simulink model "VCU10"  (R2021b)
settings: Solver=FixedStepDiscrete  StartTime=0.0  StopTime=10.0  FixedStep=0.01  RelTol=1e-3
undefined symbols (not defined in the file): F, T
libraries: simulink x149, hdlsllib x90, spsEdgeDetectorLib x2
(part 1 of 3)
settings Model: DataDictionary=VCU10DB.sldd  Creator=icemi  LastModifiedBy=icemi
settings OptimizationCC: DefaultParameterBehavior=Inlined  EnhancedBackFolding=on  PassReuseOutputArgsAs=Individual arguments  ZeroExternalMemoryAtStartup=off  ZeroInternalMemoryAtStartup=off  OptimizeBlockOrder=speed  DifferentSizesBufferReuse=on  OptimizationCustomize=off  EfficientTunableParamExpr=on
settings DebuggingCC: ParameterTunabilityLossMsg=error
settings HardwareCC: ProdBitPerPointer=32  ProdBitPerSizeT=32  ProdBitPerPtrDiffT=32  ProdLargestAtomicInteger=Long  ProdLargestAtomicFloat=Double  ProdWordSize=32  ProdHWDeviceType=ARM Compatible->ARM Cortex-M
settings SFSimCC: MATLABDynamicMemAlloc=off
settings RTWCC: Description=Embedded Coder  SystemTargetFile=ert.tlc  GenCodeOnly=on  TemplateMakefile=ert_default_tmf  CheckMdlBeforeBuild=Warning
settings CodeAppCC: ForceParamTrailComments=on  IgnoreCustomStorageClasses=off  OperatorAnnotations=on  SimulinkDataObjDesc=on  SFDataObjDesc=on  InsertBlockDesc=on
settings ERTTargetCC: TargetLangStandard=C99 (ISO)  GenerateSampleERTMain=on  ERTCustomFileBanners=off  InlinedParameterPlacement=NonHierarchical  ERTCustomFileTemplate=example_file_process.tlc

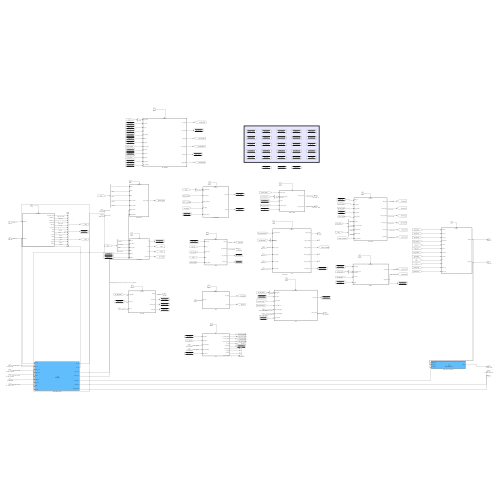
[thumbnail: Simulink's stored preview of the top-level diagram]
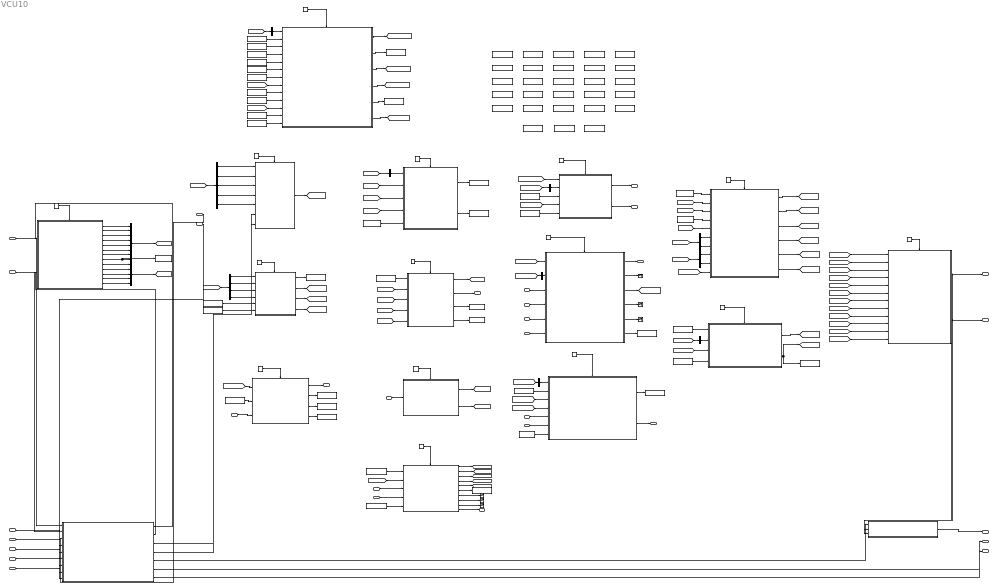
== system VCU10 ==
  note: 等待油压数据
  note: 内存
  note: VCU发送状态机运行状态以及无人任务结束，接收无人任务选择
  model_hin : Inport
  model_ain : Inport  Port=2
  wlspd_fsensor : Inport  Port=3
  wlspd_hsensor : Inport  Port=4
  AMI_Tx : Inport  Port=5
  ESP_T_01 : Inport  Port=6
  ESP_T_03 : Inport  Port=7
  ESP_T_06 : Inport  Port=8
  ESP_T_07 : Inport  Port=9
  canb_epssendmsg1 : Inport  Port=10
  canb_epssendmsg2 : Inport  Port=11
  res_msg : Inport  Port=12
  canb_ipctsmsg1 : Inport  Port=13
  canb_ipctsmsg2 : Inport  Port=14
  vcu_dbg_control : Inport  Port=15  OutDataTypeStr=uint8  PortDimensions=8
  vcu_dbg_pedal_adc : Inport  Port=16  OutDataTypeStr=uint8  PortDimensions=8
  vcu_dbg_air_wheel : Inport  Port=17  OutDataTypeStr=uint8  PortDimensions=8
  vcu_dbg_digital : Inport  Port=18  OutDataTypeStr=uint8  PortDimensions=8
  vcu_dbg_rx_count : Inport  Port=19  OutDataTypeStr=uint8  PortDimensions=4
  10ms{,1..4,6..13} (13 alike) : simulink/Ports & Subsystems/Function-Call Generator  sample_time=0.01  numberOfIterations=1  DisallowWideOutput=off
  AMI_CAN : Subsystem  TreatAsAtomicUnit=on
  ASB_Selfcheck : Subsystem  TreatAsAtomicUnit=on
  AS_Stateflow : Subsystem  TreatAsAtomicUnit=on
  Ain Bus Creator : BusCreator  Inputs=5
  Bus Selector : BusSelector  OutputSignals=apps1,apps2,brkps,airprs1,airprs2
  Bus Selector1 : BusSelector  OutputSignals=di8_side,run_button,tsms,di8_cockpit
  Bus Selector2 : BusSelector  OutputSignals=ebs_driver_check
  Bus Selector3 : BusSelector  OutputSignals=brake_flag
  Bus Selector4 : BusSelector  OutputSignals=steering_flag
  Bus Selector5 : BusSelector  OutputSignals=manual_driving_flag
  Bus Selector6 : BusSelector  OutputSignals=asms
  Bus Selector7 : BusSelector  OutputSignals=res_stop,res_communication
  Bus Selector8 : BusSelector  OutputSignals=as_emergency_flag
  Bus Selector9 : BusSelector  OutputSignals=shutdown_s,shutdown_e
  Buzzer : Subsystem  TreatAsAtomicUnit=on
  DBC_Debug_Select : MATLAB Function  TreatAsAtomicUnit=on
  DBC_Debug_StatusPack : MATLAB Function  TreatAsAtomicUnit=on
  Data Store Memory : DataStoreMemory  DataStoreName=brkmotor_check  WriteAfterWriteMsg=warning  ShowAdditionalParam=off
  Data Store Memory1 : DataStoreMemory  DataStoreName=asb_check  WriteAfterWriteMsg=warning  ShowAdditionalParam=off
  Data Store Memory10 : DataStoreMemory  DataStoreName=as_ready_flag  WriteAfterWriteMsg=warning  ShowAdditionalParam=off
  Data Store Memory11 : DataStoreMemory  DataStoreName=ts  WriteAfterWriteMsg=warning  ShowAdditionalParam=off
  Data Store Memory12 : DataStoreMemory  DataStoreName=r2d_warning  WriteAfterWriteMsg=warning  ShowAdditionalParam=off
  Data Store Memory13 : DataStoreMemory  DataStoreName=ts_flag  WriteAfterWriteMsg=warning  ShowAdditionalParam=off
  Data Store Memory14 : DataStoreMemory  DataStoreName=steer_return  WriteAfterWriteMsg=warning  ShowAdditionalParam=off
  Data Store Memory15 : DataStoreMemory  DataStoreName=as_off_flag  WriteAfterWriteMsg=warning  ShowAdditionalParam=off
  Data Store Memory16 : DataStoreMemory  DataStoreName=as_emergency_flag  WriteAfterWriteMsg=warning  ShowAdditionalParam=off
  Data Store Memory17 : DataStoreMemory  DataStoreName=as_driving_flag  WriteAfterWriteMsg=warning  ShowAdditionalParam=off
  Data Store Memory18 : DataStoreMemory  DataStoreName=r2d_flag  WriteAfterWriteMsg=warning  ShowAdditionalParam=off
  Data Store Memory19 : DataStoreMemory  DataStoreName=as_finished_flag  WriteAfterWriteMsg=warning  ShowAdditionalParam=off
  Data Store Memory2 : DataStoreMemory  DataStoreName=ebs_working  WriteAfterWriteMsg=warning  ShowAdditionalParam=off
  Data Store Memory20 : DataStoreMemory  DataStoreName=ebs_warning  WriteAfterWriteMsg=warning  ShowAdditionalParam=off
  Data Store Memory21 : DataStoreMemory  DataStoreName=task_finish  WriteAfterWriteMsg=warning  ShowAdditionalParam=off
  Data Store Memory22 : DataStoreMemory  DataStoreName=ipc_astask  WriteAfterWriteMsg=warning  ShowAdditionalParam=off
  Data Store Memory23 : DataStoreMemory  DataStoreName=ami_astask  WriteAfterWriteMsg=warning  ShowAdditionalParam=off
  Data Store Memory24 : DataStoreMemory  DataStoreName=oilprs_frsensordata  WriteAfterWriteMsg=warning  ShowAdditionalParam=off
  Data Store Memory25 : DataStoreMemory  DataStoreName=inspection_flag  WriteAfterWriteMsg=warning  ShowAdditionalParam=off
  Data Store Memory26 : DataStoreMemory  DataStoreName=astask_flag  WriteAfterWriteMsg=warning  ShowAdditionalParam=off
  Data Store Memory27 : DataStoreMemory  DataStoreName=as_flag  WriteAfterWriteMsg=warning  ShowAdditionalParam=off
  Data Store Memory3 : DataStoreMemory  DataStoreName=brake_on  WriteAfterWriteMsg=warning  ShowAdditionalParam=off
  Data Store Memory4 : DataStoreMemory  DataStoreName=ebs_check  WriteAfterWriteMsg=warning  ShowAdditionalParam=off
  Data Store Memory5 : DataStoreMemory  DataStoreName=steering_flag  WriteAfterWriteMsg=warning  ShowAdditionalParam=off
  Data Store Memory6 : DataStoreMemory  DataStoreName=brake_flag  WriteAfterWriteMsg=warning  ShowAdditionalParam=off
  Data Store Memory7 : DataStoreMemory  DataStoreName=manual_driving_flag  WriteAfterWriteMsg=warning  ShowAdditionalParam=off
  Data Store Memory8 : DataStoreMemory  DataStoreName=ebs_system_flag  WriteAfterWriteMsg=warning  ShowAdditionalParam=off
  Data Store Memory9 : DataStoreMemory  DataStoreName=steer_zero  WriteAfterWriteMsg=warning  ShowAdditionalParam=off
  Data Store Read : DataStoreRead  DataStoreName=brkmotor_check  IndexOptions=Index vector (dialog)  Indices=1  OutputSizes=1
  Data Store Read1 : DataStoreRead  DataStoreName=asb_check  IndexOptions=Index vector (dialog)  Indices=1  OutputSizes=1
  Data Store Read10 : DataStoreRead  DataStoreName=steer_zero  IndexOptions=Index vector (dialog)  Indices=1  OutputSizes=1
  Data Store Read11 : DataStoreRead  DataStoreName=ebs_warning  IndexOptions=Index vector (dialog)  Indices=1  OutputSizes=1
  Data Store Read12 : DataStoreRead  DataStoreName=task_finish  IndexOptions=Index vector (dialog)  Indices=1  OutputSizes=1
  Data Store Read13 : DataStoreRead  DataStoreName=brake_on  IndexOptions=Index vector (dialog)  Indices=1  OutputSizes=1
  Data Store Read14 : DataStoreRead  DataStoreName=inspection_flag  IndexOptions=Index vector (dialog)  Indices=1  OutputSizes=1
  Data Store Read15 : DataStoreRead  DataStoreName=ts  IndexOptions=Index vector (dialog)  Indices=1  OutputSizes=1
  Data Store Read16 : DataStoreRead  DataStoreName=astask_flag  IndexOptions=Index vector (dialog)  Indices=1  OutputSizes=1
  Data Store Read17 : DataStoreRead  DataStoreName=ipc_astask  IndexOptions=Index vector (dialog)  Indices=1  OutputSizes=1
  Data Store Read18 : DataStoreRead  DataStoreName=task_finish  IndexOptions=Index vector (dialog)  Indices=1  OutputSizes=1
  Data Store Read19 : DataStoreRead  DataStoreName=steer_return  IndexOptions=Index vector (dialog)  Indices=1  OutputSizes=1
  Data Store Read2 : DataStoreRead  DataStoreName=steer_return  IndexOptions=Index vector (dialog)  Indices=1  OutputSizes=1
  Data Store Read20 : DataStoreRead  DataStoreName=inspection_flag  IndexOptions=Index vector (dialog)  Indices=1  OutputSizes=1
  Data Store Read{21..24} (4 alike) : DataStoreRead  DataStoreName=as_flag  IndexOptions=Index vector (dialog)  Indices=1  OutputSizes=1
  Data Store Read3 : DataStoreRead  DataStoreName=r2d_warning  IndexOptions=Index vector (dialog)  Indices=1  OutputSizes=1
  Data Store Read4 : DataStoreRead  DataStoreName=ebs_check  IndexOptions=Index vector (dialog)  Indices=1  OutputSizes=1
  Data Store Read5 : DataStoreRead  DataStoreName=brake_on  IndexOptions=Index vector (dialog)  Indices=1  OutputSizes=1
  Data Store Read6 : DataStoreRead  DataStoreName=ts  IndexOptions=Index vector (dialog)  Indices=1  OutputSizes=1
  Data Store Read7 : DataStoreRead  DataStoreName=ebs_working  IndexOptions=Index vector (dialog)  Indices=1  OutputSizes=1
  Data Store Read8 : DataStoreRead  DataStoreName=brake_on  IndexOptions=Index vector (dialog)  Indices=1  OutputSizes=1
  Data Store Read9 : DataStoreRead  DataStoreName=asb_check  IndexOptions=Index vector (dialog)  Indices=1  OutputSizes=1
  Data Store Write : DataStoreWrite  DataStoreName=asb_check  IndexOptions=Index vector (dialog)  Indices=1  OutputSizes=1
  Data Store Write1 : DataStoreWrite  DataStoreName=ebs_working  IndexOptions=Index vector (dialog)  Indices=1  OutputSizes=1
  Data Store Write10 : DataStoreWrite  DataStoreName=inspection_flag  IndexOptions=Index vector (dialog)  Indices=1  OutputSizes=1
  Data Store Write11 : DataStoreWrite  DataStoreName=task_finish  IndexOptions=Index vector (dialog)  Indices=1  OutputSizes=1
  Data Store Write12 : DataStoreWrite  DataStoreName=ami_astask  IndexOptions=Index vector (dialog)  Indices=1  OutputSizes=1
  Data Store Write13 : DataStoreWrite  DataStoreName=astask_flag  IndexOptions=Index vector (dialog)  Indices=1  OutputSizes=1
  Data Store Write14 : DataStoreWrite  DataStoreName=as_flag  IndexOptions=Index vector (dialog)  Indices=1  OutputSizes=1
  Data Store Write2 : DataStoreWrite  DataStoreName=brake_on  IndexOptions=Index vector (dialog)  Indices=1  OutputSizes=1
  Data Store Write3 : DataStoreWrite  DataStoreName=ebs_check  IndexOptions=Index vector (dialog)  Indices=1  OutputSizes=1
  Data Store Write4 : DataStoreWrite  DataStoreName=brkmotor_check  IndexOptions=Index vector (dialog)  Indices=1  OutputSizes=1
  Data Store Write5 : DataStoreWrite  DataStoreName=steer_zero  IndexOptions=Index vector (dialog)  Indices=1  OutputSizes=1
  Data Store Write6 : DataStoreWrite  DataStoreName=ts  IndexOptions=Index vector (dialog)  Indices=1  OutputSizes=1
  Data Store Write7 : DataStoreWrite  DataStoreName=ebs_warning  IndexOptions=Index vector (dialog)  Indices=1  OutputSizes=1
  Data Store Write8 : DataStoreWrite  DataStoreName=r2d_warning  IndexOptions=Index vector (dialog)  Indices=1  OutputSizes=1
  Data Store Write9 : DataStoreWrite  DataStoreName=steer_return  IndexOptions=Index vector (dialog)  Indices=1  OutputSizes=1
  EBS : Subsystem  TreatAsAtomicUnit=on
  EPS : Subsystem
  ESP : Subsystem
  Function-Call Generator : simulink/Ports & Subsystems/Function-Call Generator  sample_time=0.01  numberOfIterations=1  DisallowWideOutput=off
  Function-Call Generator1 : simulink/Ports & Subsystems/Function-Call Generator  sample_time=0.01  numberOfIterations=1  DisallowWideOutput=off
  Hin Bus Creator : BusCreator  Inputs=8
  IPC : Subsystem  TreatAsAtomicUnit=on
  Input_Convert : Subsystem  TreatAsAtomicUnit=on
  LED_Control : Subsystem
  Motor_Control : Subsystem  TreatAsAtomicUnit=on
  Output_Convert : Subsystem  TreatAsAtomicUnit=on
  Res : Subsystem
  Sensor_Signal : Subsystem  TreatAsAtomicUnit=on
  TS_Activation : Subsystem  TreatAsAtomicUnit=on
  Terminator{,1..5} (6 alike) : Terminator
  model_lox : Outport
  model_hox : Outport  Port=2
  ebs_watchdog : Outport  Port=3
  AMI_RX : Outport  Port=4
  ESP_R_00 : Outport  Port=5
  canb_epsmsg : Outport  Port=6
  canb_ipcrxmsg : Outport  Port=7
  cana_motor_cmd : Outport  Port=8
  cana_motor_cmd3 : Outport  Port=9
  vcu_dbg_status : Outport  Port=10  OutDataTypeStr=uint8  PortDimensions=8
  vcu_dbg_pedal_echo : Outport  Port=11  OutDataTypeStr=uint8  PortDimensions=8
  vcu_dbg_air_wheel_echo : Outport  Port=12  OutDataTypeStr=uint8  PortDimensions=8
  wires:
  Function-Call Generator/1 -> Input_Convert/Trigger
  Input_Convert/1(ebs_driver_check) -> Hin Bus Creator/1  "ebs_driver_check"
  Input_Convert/2(shutdown_s) -> Hin Bus Creator/2  "shutdown_s"
  Input_Convert/3(shutdown_e) -> Hin Bus Creator/3  "shutdown_e"
  Input_Convert/4(di8_cockpit) -> Hin Bus Creator/4  "di8_cockpit"
  Input_Convert/5(di8_side) -> Hin Bus Creator/5  "di8_side"
  Input_Convert/6(run_button) -> Hin Bus Creator/6  "run_button"
  Input_Convert/7(tsms) -> Hin Bus Creator/7  "tsms"
  Input_Convert/8(asms) -> Data Store Write14/1, Hin Bus Creator/8  "asms"
  Input_Convert/9(apps1) -> Ain Bus Creator/1  "apps1"
  Input_Convert/10(apps2) -> Ain Bus Creator/2  "apps2"
  Input_Convert/11(brkps) -> Ain Bus Creator/3  "brkps"
  Input_Convert/12(airprs1) -> Ain Bus Creator/4  "airprs1"
  Input_Convert/13(airprs2) -> Ain Bus Creator/5  "airprs2"
  Hin Bus Creator/1 -> [Hin]
  Ain Bus Creator/1 -> [Ain]
  Function-Call Generator1/1 -> Output_Convert/Trigger
  [led_brake] -> Output_Convert/1(led_brake)
  [led_assi_y] -> Output_Convert/2(led_assi_y)
  [led_assi_b] -> Output_Convert/3(led_assi_b)
  [led_ebserror] -> Output_Convert/4(led_ebserror)
  [res_err] -> Output_Convert/5(res_error)
  [ebs_trig] -> Output_Convert/6(ebs_trig)
  [led_bmserr] -> Output_Convert/7(led_bmserr)
  [led_imderr] -> Output_Convert/8(led_imderr)
  [di8] -> Output_Convert/9(di8)
  [run] -> Output_Convert/10(run)
  [buzzer_r2d] -> Output_Convert/11(buzzer_r2d)
  [buzzer_ebs] -> Output_Convert/12(buzzer_ebs)
  Output_Convert/1(model_lox) -> model_lox/1, DBC_Debug_StatusPack/2(model_lox)
  Output_Convert/2(model_hox) -> model_hox/1, DBC_Debug_StatusPack/3(model_hox)
  10ms/1 -> Sensor_Signal/Trigger
  Sensor_Signal/1(sensor_signal) -> [sensor_signal]
  [Ain] -> Bus Selector/1
  Bus Selector/1 -> Sensor_Signal/1(apps1)  "<apps1>"
  Bus Selector/2 -> Sensor_Signal/2(apps2)  "<apps2>"
  Bus Selector/3 -> Sensor_Signal/3(brkps)  "<brkps>"
  Bus Selector/4 -> Sensor_Signal/4(airprs_sensor1)  "<airprs1>"
  Bus Selector/5 -> Sensor_Signal/5(airprs_sensor2)  "<airprs2>"
  TS_Activation/1(ts) -> Data Store Write6/1
  TS_Activation/3(run) -> [run]
  TS_Activation/2(di8) -> [di8]
  Data Store Read5/1 -> TS_Activation/6(brake_on)
  TS_Activation/4(ts_warning) -> [ts_warning]
  10ms1/1 -> TS_Activation/Trigger
  [Hin] -> Bus Selector1/1
  Bus Selector1/1 -> TS_Activation/1(di8_out)  "<di8_side>"
  Bus Selector1/2 -> TS_Activation/2(run_button)  "<run_button>"
  Bus Selector1/3 -> TS_Activation/3(tsms_button)  "<tsms>"
  Bus Selector1/4 -> TS_Activation/4(di8_in)  "<di8_cockpit>"
  ASB_Selfcheck/2(brake_on) -> Data Store Write2/1
  [sensor_signal] -> ASB_Selfcheck/2(sensor_signal)
  [res_signal] -> ASB_Selfcheck/4(res_signal)
  Data Store Read/1 -> ASB_Selfcheck/5(brkmotor_check)
  [ESP_T_03signal] -> ASB_Selfcheck/3(ESP_T_03signal)
  ASB_Selfcheck/1(asb_check) -> Data Store Write/1
  10ms3/1 -> ASB_Selfcheck/Trigger
  [Hin] -> Bus Selector2/1
  Bus Selector2/1 -> ASB_Selfcheck/1(ebs_drivercheck)  "<ebs_driver_check>"
  10ms7/1 -> EBS/Trigger
  Data Store Read1/1 -> EBS/1(asb_check)
  [as_ebs_trig] -> EBS/3(as_ebs_trig)
  [ipc_err] -> EBS/2(ipc_err)
  EBS/2(ebs_watchdog) -> ebs_watchdog/1  "ebs_watchdog"
  EBS/1(ebs_trig) -> [ebs_trig]  "ebs_trig"
  [sensor_signal] -> EBS/5(sensor_signal)
  [Hin] -> EBS/4(Hin)
  EBS/3(ebs_working) -> Data Store Write1/1
  EBS/4(ebs_check) -> Data Store Write3/1
  AMI_CAN/1(AMI_RX) -> AMI_RX/1  "AMI_Rx"
  [as_flag_state] -> AMI_CAN/1(as_flag_state)
  AMI_Tx/1 -> AMI_CAN/3(AMI_Tx)  "AMI_Tx"
  10ms13/1 -> AMI_CAN/Trigger
  AMI_CAN/2(ami_astask) -> Data Store Write12/1
  Data Store Read12/1 -> AMI_CAN/2(task_finish)
  [as_flag_state] -> Bus Selector3/1
  ESP_T_06/1 -> ESP/5(canb_esp_t06)  "ESP_T_06"
  ESP/5(ESP_T_07signal) -> Terminator3/1
  ESP_T_01/1 -> ESP/3(canb_esp_t01)  "ESP_T_01"
  ESP_T_03/1 -> ESP/4(canb_esp_t03)  "ESP_T_03"
  Bus Selector3/1 -> ESP/2(brake_flag)  "<brake_flag>"
  ESP/1(canb_esp_r00) -> ESP_R_00/1
  ESP/2(ESP_T_01sigal) -> Terminator/1
  ESP/3(ESP_T_03signal) -> [ESP_T_03signal]
  ESP/6(brkmotor_check) -> Data Store Write4/1
  ESP/4(ESP_T_06signal) -> Terminator2/1
  ESP_T_07/1 -> ESP/6(canb_esp_t07)  "ESP_T_07"
  [ipc_esp_pressure] -> ESP/1(ipc_esp_pressure)
  10ms8/1 -> ESP/Trigger
  Data Store Read2/1 -> EPS/2(steer_return)
  Data Store Read14/1 -> EPS/7(ami_inspection)
  EPS/2(canb_epsmsg) -> canb_epsmsg/1  "canb_epsmsg"
  EPS/1(steer_zero) -> Data Store Write5/1
  [as_flag_state] -> Bus Selector4/1
  [ipc_eps_angle] -> EPS/3(ipc_eps_angle)
  canb_epssendmsg2/1 -> EPS/6(canb_epssendmsg2)  "canb_epssendmsg2"
  canb_epssendmsg1/1 -> EPS/5(canb_epssendmsg1)  "canb_epssendmsg1"
  Bus Selector4/1 -> EPS/1(steering_flag)  "<steering_flag>"
  10ms9/1 -> EPS/Trigger
  [ipc_eps_velocity] -> EPS/4(ipc_eps_velocity)
  res_msg/1 -> Res/1(res_msg)  "res_msg"
  10ms10/1 -> Res/Trigger
  Res/2(res_error) -> [res_err]  "res_error"
  Res/1(res_signal) -> [res_signal]
  [res_signal] -> IPC/2(res_signal)
  IPC/3(ipc_eps_angle) -> [ipc_eps_angle]
  IPC/5(ipc_err) -> [ipc_err]
  IPC/1(ipc_esp_pressure) -> [ipc_esp_pressure]
  canb_ipctsmsg1/1 -> IPC/3(canb_ipctsmsg1)  "canb_ipctsmsg1"
  canb_ipctsmsg2/1 -> IPC/4(canb_ipctsmsg2)  "canb_ipctsmsg2"
  IPC/10(canb_ipcrxmsg) -> canb_ipcrxmsg/1  "canb_ipcrxmsg"
  IPC/6(task_finish) -> Data Store Write11/1
  IPC/8(ipc_lspd) -> Terminator4/1
  IPC/4(ipc_eps_velocity) -> [ipc_eps_velocity]
  IPC/9(ipc_hspd) -> Terminator5/1
  Data Store Read19/1 -> IPC/5(steer_return)
  Data Store Read17/1 -> IPC/1(ipc_astask)
  IPC/2(ipc_motor_torque) -> [ipc_motor_torque]
  10ms11/1 -> IPC/Trigger
  IPC/7(ipc_heartbeat) -> Terminator1/1
  Motor_Control/1(cana_motor_cmd) -> cana_motor_cmd/1  "cana_motor_cmd"
  [sensor_signal] -> Motor_Control/1(sensor_signal)
  [ipc_motor_torque] -> Motor_Control/4(ipc_motor_torque)
  [as_flag_state] -> Bus Selector5/1
  Data Store Read21/1 -> Motor_Control/3(as_flag)
  Bus Selector5/1 -> Motor_Control/2(manual_driving_flag)  "<manual_driving_flag>"
  Motor_Control/2(cana_motor_cmd3) -> cana_motor_cmd3/1  "cana_motor_cmd3"
  Data Store Read15/1 -> Motor_Control/5(ts)
  10ms4/1 -> Motor_Control/Trigger
  Data Store Read10/1 -> AS_Stateflow/10(steer_zero)
  AS_Stateflow/5(steer_return) -> Data Store Write9/1
  AS_Stateflow/2(r2d_warning) -> Data Store Write8/1
  Data Store Read20/1 -> AS_Stateflow/13(ami_inspection)
  [sensor_signal] -> AS_Stateflow/8(sensor_signal)
  Data Store Read8/1 -> AS_Stateflow/6(brake_on)
  Data Store Read11/1 -> AS_Stateflow/12(ebs_warning)
  AS_Stateflow/6(as_flag_state) -> [as_flag_state]
  [res_signal] -> AS_Stateflow/11(res_signal)
  10ms6/1 -> AS_Stateflow/Trigger
  AS_Stateflow/4(as_led_yellow) -> [as_led_yellow]
  Data Store Read9/1 -> AS_Stateflow/7(asb_check)
  Data Store Read6/1 -> AS_Stateflow/4(ts)
  Data Store Read7/1 -> AS_Stateflow/5(ebs_working)
  Data Store Read18/1 -> AS_Stateflow/9(task_finish)
  Data Store Read16/1 -> AS_Stateflow/3(as_task)
  Data Store Read4/1 -> AS_Stateflow/2(ebs_check)
  AS_Stateflow/1(as_ebs_trig) -> [as_ebs_trig]
  AS_Stateflow/3(as_led_blue) -> [as_led_blue]
  [Hin] -> Bus Selector6/1
  Bus Selector6/1 -> AS_Stateflow/1(asms_button)  "<asms>"
  LED_Control/3(led_assi_yellow) -> [led_assi_y]  "led_assi_yellow"
  [ESP_T_03signal] -> LED_Control/10(ESP_T_03signal)
  Bus Selector7/1 -> LED_Control/6(res_stop)  "<res_stop>"
  [sensor_signal] -> LED_Control/5(sensor_signal)
  Bus Selector7/2 -> LED_Control/7(res_communication)  "<res_communication>"
  Data Store Read13/1 -> LED_Control/1(brake_on)
  Data Store Read22/1 -> LED_Control/4(asms_button)
  10ms2/1 -> LED_Control/Trigger
  [as_led_yellow] -> LED_Control/3(as_led_yellow)
  LED_Control/4(led_ebs_error) -> [led_ebserror]  "led_ebs_error"
  LED_Control/2(led_assi_blue) -> [led_assi_b]  "led_assi_blue"
  [as_led_blue] -> LED_Control/2(as_led_blue)
  LED_Control/1(led_brake) -> [led_brake]  "led_brake"
  [res_signal] -> Bus Selector7/1
  Data Store Read3/1 -> Buzzer/1(r2d_warning)
  Buzzer/2(ebs_buzzer) -> [buzzer_ebs], Data Store Write7/1  "ebs_buzzer"
  Bus Selector8/1 -> Buzzer/2(as_emergency_flag)  "<as_emergency_flag>"
  [ts_warning] -> Buzzer/3(ts_warning)
  [as_flag_state] -> Bus Selector8/1
  10ms12/1 -> Buzzer/Trigger
  Buzzer/1(r2d_buzzer) -> [buzzer_r2d]  "r2d_buzzer"
  AMI_CAN/3(inspection_flag) -> Data Store Write10/1
  AMI_CAN/4(astask_flag) -> Data Store Write13/1
  Data Store Read23/1 -> TS_Activation/5(as_flag)
  Data Store Read24/1 -> Buzzer/4(as_flag)
  LED_Control/5(led_imderr) -> [led_imderr]  "led_imd_error"
  LED_Control/6(led_bmserr) -> [led_bmserr]  "led_bms_error"
  [Hin] -> Bus Selector9/1
  Bus Selector9/1 -> LED_Control/8(Shutdown_Start)  "<shutdown_s>"
  Bus Selector9/2 -> LED_Control/9(Shutdown_End)  "<shutdown_e>"
  model_hin/1 -> DBC_Debug_Select/1(hin_hw)  "model_hin"
  DBC_Debug_Select/1(hin_sel) -> Input_Convert/1(model_hin)
  model_ain/1 -> DBC_Debug_Select/2(ain_hw)  "model_ain"
  DBC_Debug_Select/2(ain_sel) -> Input_Convert/2(model_ain)
  wlspd_fsensor/1 -> DBC_Debug_Select/3(wheel_f_hw)  "wlspd_fsensor"
  DBC_Debug_Select/3(wheel_f_sel) -> Sensor_Signal/6(wlspd_fsensor)
  wlspd_hsensor/1 -> DBC_Debug_Select/4(wheel_h_hw)  "wlspd_hsensor"
  DBC_Debug_Select/4(wheel_h_sel) -> Sensor_Signal/7(wlspd_hsensor)
  vcu_dbg_control/1 -> DBC_Debug_Select/5(control)  "vcu_dbg_control"
  vcu_dbg_pedal_adc/1 -> DBC_Debug_Select/6(pedal_adc)  "vcu_dbg_pedal_adc"
  vcu_dbg_air_wheel/1 -> DBC_Debug_Select/7(air_wheel)  "vcu_dbg_air_wheel"
  vcu_dbg_digital/1 -> DBC_Debug_Select/8(digital)  "vcu_dbg_digital"
  vcu_dbg_rx_count/1 -> DBC_Debug_Select/9(rx_count)  "vcu_dbg_rx_count"
  DBC_Debug_Select/5(status_base) -> DBC_Debug_StatusPack/1(status_base)
  DBC_Debug_StatusPack/1(status) -> vcu_dbg_status/1
  DBC_Debug_Select/6(pedal_echo) -> vcu_dbg_pedal_echo/1
  DBC_Debug_Select/7(air_wheel_echo) -> vcu_dbg_air_wheel_echo/1

== system VCU10/AMI_CAN ==
  as_flag_state : Inport
  task_finish : Inport  Port=2
  AMI_Tx : Inport  Port=3
  function : TriggerPort  TriggerType=function-call  VariantControl=(inherit)
  AMI_Receivemsg : Subsystem
  AMI_Transmitmsg : Subsystem
  Compare To Constant : simulink/Logic and Bit Operations/Compare To Constant  relop===  const=5  OutDataTypeStr=boolean
  Compare To Constant1 : simulink/Logic and Bit Operations/Compare To Constant  relop=>  const=0  OutDataTypeStr=boolean
  AMI_RX : Outport
  ami_astask : Outport  Port=2
  inspection_flag : Outport  Port=3
  astask_flag : Outport  Port=4
  wires:
  AMI_Receivemsg/1(ami_astask) -> Compare To Constant1/1, Compare To Constant/1, ami_astask/1
  AMI_Tx/1 -> AMI_Receivemsg/1(AMI_Tx)
  as_flag_state/1 -> AMI_Transmitmsg/1(as_flag_state)
  task_finish/1 -> AMI_Transmitmsg/2(task_finish)
  AMI_Transmitmsg/1(AMI_RX) -> AMI_RX/1
  Compare To Constant/1 -> inspection_flag/1
  Compare To Constant1/1 -> astask_flag/1

== system VCU10/ASB_Selfcheck ==
  note: 制动相关压力是否支持正常工作
  note: EBS驱动板上电检查
  ebs_drivercheck : Inport
  sensor_signal : Inport  Port=2
  ESP_T_03signal : Inport  Port=3
  res_signal : Inport  Port=4
  brkmotor_check : Inport  Port=5
  function : TriggerPort  TriggerType=function-call  VariantControl=(inherit)
  Brake_Sensor_Check : Subsystem
  Bus Selector : BusSelector  OutputSignals=airprs_sensor1
  Bus Selector1 : BusSelector  OutputSignals=res_check
  Bus Selector2 : BusSelector  OutputSignals=oilprs_flsensor,oilprs_frsensor,oilprs_rlsensor,oilprs_rrsensor
  Logical Operator : Logic  Inputs=4  AllPortsSameDT=off  OutDataTypeStr=boolean
  asb_check : Outport
  brake_on : Outport  Port=2
  wires:
  sensor_signal/1 -> Bus Selector/1
  Bus Selector/1 -> Brake_Sensor_Check/1(airprs_sensor1)  "<airprs_sensor1>"
  ebs_drivercheck/1 -> Logical Operator/1
  brkmotor_check/1 -> Logical Operator/4
  Logical Operator/1 -> asb_check/1
  Brake_Sensor_Check/2(brake_on) -> brake_on/1
  res_signal/1 -> Bus Selector1/1
  ESP_T_03signal/1 -> Bus Selector2/1
  Bus Selector2/1 -> Brake_Sensor_Check/2(oilprs_frsensor)  "<oilprs_flsensor>"
  Bus Selector2/2 -> Brake_Sensor_Check/3(oilprs_rrsensor)  "<oilprs_frsensor>"
  Bus Selector2/3 -> Brake_Sensor_Check/4(oilprs_flsensor)  "<oilprs_rlsensor>"
  Bus Selector2/4 -> Brake_Sensor_Check/5(oilprs_rlsensor)  "<oilprs_rrsensor>"
  Bus Selector1/1 -> Logical Operator/2  "<res_check>"
  Brake_Sensor_Check/1(brksensor_check) -> Logical Operator/3

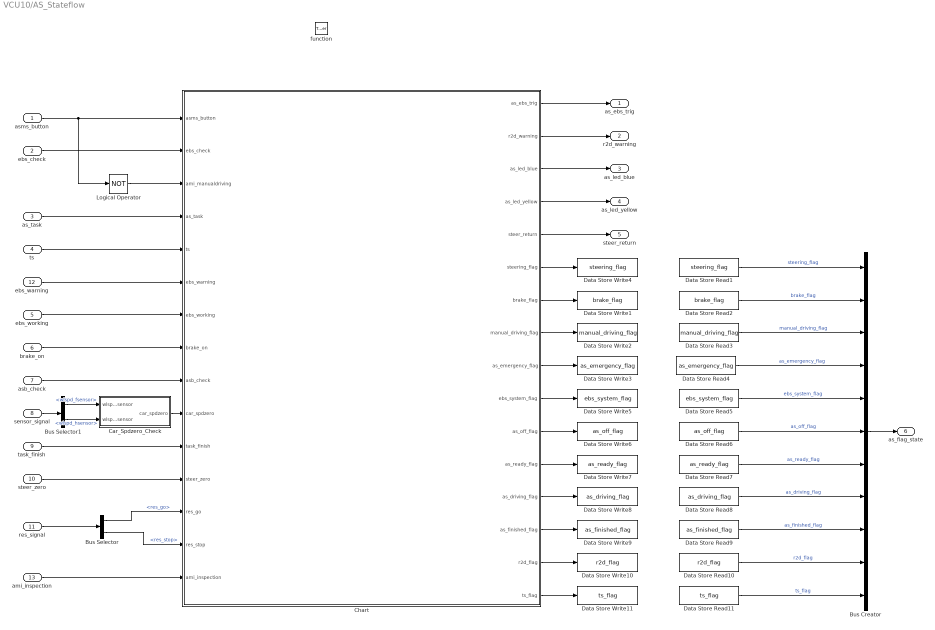
== system VCU10/AS_Stateflow ==
  asms_button : Inport
  ebs_check : Inport  Port=2
  as_task : Inport  Port=3
  ts : Inport  Port=4
  ebs_working : Inport  Port=5
  brake_on : Inport  Port=6
  asb_check : Inport  Port=7
  sensor_signal : Inport  Port=8
  task_finish : Inport  Port=9
  steer_zero : Inport  Port=10
  res_signal : Inport  Port=11
  ebs_warning : Inport  Port=12
  ami_inspection : Inport  Port=13
  function : TriggerPort  TriggerType=function-call  VariantControl=(inherit)
  Bus Creator : BusCreator  Inputs=11
  Bus Selector : BusSelector  OutputSignals=res_go,res_stop
  Bus Selector1 : BusSelector  OutputSignals=wlspd_fsensor,wlspd_hsensor
  Car_Spdzero_Check : Subsystem
  Chart : Stateflow chart  TreatAsAtomicUnit=on
      settings: PortSchema="{\"entries\":[{\"content\":{\"sides\":[{\"content\":{\"connectorIds\":[\"In1\",\"In2\",\"In3\",\"In4\",\"In5\",\"In6\",\"In7\",\"In8\",\"In9\",\"In10\",\"In11\",\"In13\",\"In12\",\"In14\",\"In15\"]},\"type\":\"ConnectorPlacement.EquallySpacedRectSide\",\"uuid\":\"5ff7b962-0009-43e2-919e-affd8aae6d9f\"},{\"content\":{\"connectorIds\":[\"Out1\",\"Out2\",\"Out3\",\"Out4\",\"Out5\",\"Out6\",\"Out7\",\"Out8\",\"Out9\",\"Out10\",\"Out11\",\"Out12\",\"Out13\",\"Out14\",\"Out15\",\"Out16\"],\"side\":\"RIGHT\"},\"type\":\"ConnectorPlacement.EquallySpacedRectSide\",\"uuid\":\"8fbd6d23-6f6b-4ff9-8347-09da63d88237\"},{\"content\":{\"side\":\"TOP\"},\"type\":\"ConnectorPlacement.EquallySpacedRectSide\",\"uuid\":\"5115a408-a5f8-47e8-8fa4-cf60e643eb64\"}]},\"type\":\"ConnectorPlacement.EquallySpacedConnector\",\"uuid\":\"6f9469b9-2522-48d3-80b2-5e824d353f63\"}],\"packageUris\":[\"http://schema.mathworks.com/mf0/Connector/R2020b\"],\"version\":\"1.0\"}"
  Data Store Read1 : DataStoreRead  DataStoreName=steering_flag  IndexOptions=Index vector (dialog)  Indices=1  OutputSizes=1
  Data Store Read10 : DataStoreRead  DataStoreName=r2d_flag  IndexOptions=Index vector (dialog)  Indices=1  OutputSizes=1
  Data Store Read11 : DataStoreRead  DataStoreName=ts_flag  IndexOptions=Index vector (dialog)  Indices=1  OutputSizes=1
  Data Store Read2 : DataStoreRead  DataStoreName=brake_flag  IndexOptions=Index vector (dialog)  Indices=1  OutputSizes=1
  Data Store Read3 : DataStoreRead  DataStoreName=manual_driving_flag  IndexOptions=Index vector (dialog)  Indices=1  OutputSizes=1
  Data Store Read4 : DataStoreRead  DataStoreName=as_emergency_flag  IndexOptions=Index vector (dialog)  Indices=1  OutputSizes=1
  Data Store Read5 : DataStoreRead  DataStoreName=ebs_system_flag  IndexOptions=Index vector (dialog)  Indices=1  OutputSizes=1
  Data Store Read6 : DataStoreRead  DataStoreName=as_off_flag  IndexOptions=Index vector (dialog)  Indices=1  OutputSizes=1
  Data Store Read7 : DataStoreRead  DataStoreName=as_ready_flag  IndexOptions=Index vector (dialog)  Indices=1  OutputSizes=1
  Data Store Read8 : DataStoreRead  DataStoreName=as_driving_flag  IndexOptions=Index vector (dialog)  Indices=1  OutputSizes=1
  Data Store Read9 : DataStoreRead  DataStoreName=as_finished_flag  IndexOptions=Index vector (dialog)  Indices=1  OutputSizes=1
  Data Store Write1 : DataStoreWrite  DataStoreName=brake_flag  IndexOptions=Index vector (dialog)  Indices=1  OutputSizes=1
  Data Store Write10 : DataStoreWrite  DataStoreName=r2d_flag  IndexOptions=Index vector (dialog)  Indices=1  OutputSizes=1
  Data Store Write11 : DataStoreWrite  DataStoreName=ts_flag  IndexOptions=Index vector (dialog)  Indices=1  OutputSizes=1
  Data Store Write2 : DataStoreWrite  DataStoreName=manual_driving_flag  IndexOptions=Index vector (dialog)  Indices=1  OutputSizes=1
  Data Store Write3 : DataStoreWrite  DataStoreName=as_emergency_flag  IndexOptions=Index vector (dialog)  Indices=1  OutputSizes=1
  Data Store Write4 : DataStoreWrite  DataStoreName=steering_flag  IndexOptions=Index vector (dialog)  Indices=1  OutputSizes=1
  Data Store Write5 : DataStoreWrite  DataStoreName=ebs_system_flag  IndexOptions=Index vector (dialog)  Indices=1  OutputSizes=1
  Data Store Write6 : DataStoreWrite  DataStoreName=as_off_flag  IndexOptions=Index vector (dialog)  Indices=1  OutputSizes=1
  Data Store Write7 : DataStoreWrite  DataStoreName=as_ready_flag  IndexOptions=Index vector (dialog)  Indices=1  OutputSizes=1
  Data Store Write8 : DataStoreWrite  DataStoreName=as_driving_flag  IndexOptions=Index vector (dialog)  Indices=1  OutputSizes=1
  Data Store Write9 : DataStoreWrite  DataStoreName=as_finished_flag  IndexOptions=Index vector (dialog)  Indices=1  OutputSizes=1
  Logical Operator : Logic  Operator=NOT  AllPortsSameDT=off  OutDataTypeStr=boolean
  as_ebs_trig : Outport
  r2d_warning : Outport  Port=2
  as_led_blue : Outport  Port=3
  as_led_yellow : Outport  Port=4
  steer_return : Outport  Port=5
  as_flag_state : Outport  Port=6
  wires:
  ebs_check/1 -> Chart/2(ebs_check)
  as_task/1 -> Chart/4(as_task)
  ebs_working/1 -> Chart/7(ebs_working)
  brake_on/1 -> Chart/8(brake_on)
  asb_check/1 -> Chart/9(asb_check)
  task_finish/1 -> Chart/11(task_finish)
  steer_zero/1 -> Chart/13(steer_zero)
  ts/1 -> Chart/5(ts)
  Chart/1(as_ebs_trig) -> as_ebs_trig/1
  Chart/2(r2d_warning) -> r2d_warning/1
  Chart/3(as_led_blue) -> as_led_blue/1
  Chart/4(as_led_yellow) -> as_led_yellow/1
  Chart/5(steer_return) -> steer_return/1
  ebs_warning/1 -> Chart/6(ebs_warning)
  res_signal/1 -> Bus Selector/1
  Bus Selector/2 -> Chart/14(res_stop)  "<res_stop>"
  Bus Selector/1 -> Chart/12(res_go)  "<res_go>"
  sensor_signal/1 -> Bus Selector1/1
  Bus Selector1/1 -> Car_Spdzero_Check/1(wlspd_fsensor)  "<wlspd_fsensor>"
  Bus Selector1/2 -> Car_Spdzero_Check/2(wlspd_hsensor)  "<wlspd_hsensor>"
  Car_Spdzero_Check/1(car_spdzero) -> Chart/10(car_spdzero)
  Bus Creator/1 -> as_flag_state/1
  Chart/6(steering_flag) -> Data Store Write4/1
  Data Store Read1/1 -> Bus Creator/1  "steering_flag"
  Chart/7(brake_flag) -> Data Store Write1/1
  Data Store Read2/1 -> Bus Creator/2  "brake_flag"
  Chart/8(manual_driving_flag) -> Data Store Write2/1
  Data Store Read3/1 -> Bus Creator/3  "manual_driving_flag"
  Data Store Read4/1 -> Bus Creator/4  "as_emergency_flag"
  Chart/9(as_emergency_flag) -> Data Store Write3/1
  Chart/10(ebs_system_flag) -> Data Store Write5/1
  Data Store Read5/1 -> Bus Creator/5  "ebs_system_flag"
  Chart/11(as_off_flag) -> Data Store Write6/1
  Data Store Read6/1 -> Bus Creator/6  "as_off_flag"
  Chart/12(as_ready_flag) -> Data Store Write7/1
  Data Store Read7/1 -> Bus Creator/7  "as_ready_flag"
  Chart/13(as_driving_flag) -> Data Store Write8/1
  Data Store Read8/1 -> Bus Creator/8  "as_driving_flag"
  Chart/14(as_finished_flag) -> Data Store Write9/1
  Data Store Read9/1 -> Bus Creator/9  "as_finished_flag"
  Chart/15(r2d_flag) -> Data Store Write10/1
  Data Store Read10/1 -> Bus Creator/10  "r2d_flag"
  Data Store Read11/1 -> Bus Creator/11  "ts_flag"
  Chart/16(ts_flag) -> Data Store Write11/1
  ami_inspection/1 -> Chart/15(ami_inspection)
  asms_button/1 -> Logical Operator/1, Chart/1(asms_button)
  Logical Operator/1 -> Chart/3(ami_manualdriving)

== system VCU10/Buzzer ==
  r2d_warning : Inport
  as_emergency_flag : Inport  Port=2
  ts_warning : Inport  Port=3
  as_flag : Inport  Port=4
  function : TriggerPort  TriggerType=function-call  VariantControl=(inherit)
  Chart : Stateflow chart  TreatAsAtomicUnit=on
  Constant : Constant  Value=0  OutDataTypeStr=boolean
  Data Type Conversion6 : DataTypeConversion  OutDataTypeStr=boolean
  Pulse Generator : DiscretePulseGenerator  Period=100  PulseWidth=50  SampleTime=-1
  Switch : Switch  Criteria=u2 > Threshold
  Switch1 : Switch  Criteria=u2 > Threshold
  r2d_buzzer : Outport
  ebs_buzzer : Outport  Port=2
  wires:
  as_emergency_flag/1 -> Chart/1(as_emergency_flag)
  Chart/1(ebs_buzzer) -> Switch/2
  Switch/1 -> ebs_buzzer/1
  Constant/1 -> Switch/3
  Pulse Generator/1 -> Data Type Conversion6/1
  Data Type Conversion6/1 -> Switch/1
  r2d_warning/1 -> Switch1/1
  ts_warning/1 -> Switch1/3
  as_flag/1 -> Switch1/2
  Switch1/1 -> r2d_buzzer/1

== system VCU10/EBS ==
  note: 气压传感器值待定
  asb_check : Inport
  ipc_err : Inport  Port=2
  as_ebs_trig : Inport  Port=3
  Hin : Inport  Port=4
  sensor_signal : Inport  Port=5
  function : TriggerPort  TriggerType=function-call  VariantControl=(inherit)
  Bus Selector : BusSelector  OutputSignals=asms,ebs_driver_check
  Bus Selector1 : BusSelector  OutputSignals=airprs_sensor1,airprs_sensor2
  Compare To Constant : simulink/Logic and Bit Operations/Compare To Constant  relop=>=  const=6  OutDataTypeStr=boolean
  Compare To Constant1 : simulink/Logic and Bit Operations/Compare To Constant  relop=<=  const=5.5  OutDataTypeStr=boolean
  Edge Detector : spsEdgeDetectorLib/Edge Detector  model=Falling  ic=0  Ts=-1
      settings: SourceProductBaseCode=PS
  Edge Detector2 : spsEdgeDetectorLib/Edge Detector  model=Rising  ic=0  Ts=-1
      settings: SourceProductBaseCode=PS
  Logical Operator : Logic  Operator=OR  Inputs=3  AllPortsSameDT=off  OutDataTypeStr=boolean
  Logical Operator1 : Logic  AllPortsSameDT=off  OutDataTypeStr=boolean
  Logical Operator2 : Logic  AllPortsSameDT=off  OutDataTypeStr=boolean
  Logical Operator3 : Logic  Operator=NOT  AllPortsSameDT=off  OutDataTypeStr=boolean
  ebs_trig : Outport
  ebs_watchdog : Outport  Port=2
  ebs_working : Outport  Port=3
  ebs_check : Outport  Port=4
  wires:
  asb_check/1 -> Edge Detector/1
  ipc_err/1 -> Edge Detector2/1
  Edge Detector/1 -> Logical Operator/1
  Edge Detector2/1 -> Logical Operator/2
  as_ebs_trig/1 -> Logical Operator/3
  Logical Operator/1 -> ebs_trig/1
  Hin/1 -> Bus Selector/1
  Bus Selector/1 -> ebs_watchdog/1  "<asms>"
  sensor_signal/1 -> Bus Selector1/1
  Bus Selector1/1 -> Compare To Constant/1  "<airprs_sensor1>"
  Compare To Constant/1 -> Logical Operator1/2
  Logical Operator1/1 -> ebs_working/1, Logical Operator3/1
  Bus Selector/2 -> Logical Operator1/1  "<ebs_driver_check>"
  Bus Selector1/2 -> Compare To Constant1/1  "<airprs_sensor2>"
  Logical Operator3/1 -> Logical Operator2/1
  Compare To Constant1/1 -> Logical Operator2/2
  Logical Operator2/1 -> ebs_check/1

== system VCU10/EPS ==
  steering_flag : Inport
  steer_return : Inport  Port=2
  ipc_eps_angle : Inport  Port=3
  ipc_eps_velocity : Inport  Port=4
  canb_epssendmsg1 : Inport  Port=5
  canb_epssendmsg2 : Inport  Port=6
  ami_inspection : Inport  Port=7
  function : TriggerPort  TriggerType=function-call  VariantControl=(inherit)
  Bus Selector : BusSelector  OutputSignals=eps_realangle
  EPS_ReceiveMsg : Subsystem
  EPS_TransmitMsg : Subsystem
  Terminator : Terminator
  steer_zero : Outport
  canb_epsmsg : Outport  Port=2
  wires:
  steering_flag/1 -> EPS_TransmitMsg/1(steering_flag)
  steer_return/1 -> EPS_TransmitMsg/2(steer_return)
  ipc_eps_angle/1 -> EPS_TransmitMsg/3(eps_wheel_angle)
  ipc_eps_velocity/1 -> EPS_TransmitMsg/4(ipc_eps_velocity)
  EPS_TransmitMsg/1(canb_epsmsg) -> canb_epsmsg/1
  EPS_TransmitMsg/2(steer_zero) -> steer_zero/1
  canb_epssendmsg1/1 -> EPS_ReceiveMsg/1(canb_epssendmsg1)
  canb_epssendmsg2/1 -> EPS_ReceiveMsg/2(canb_epssendmsg2)
  EPS_ReceiveMsg/2(canb_epssendmsg2signal) -> Terminator/1
  EPS_ReceiveMsg/1(canb_epssendmsg1signal) -> [canb_epssendmsg1signal]
  Bus Selector/1 -> EPS_TransmitMsg/5(eps_realangle)  "<eps_realangle>"
  [canb_epssendmsg1signal] -> Bus Selector/1
  ami_inspection/1 -> EPS_TransmitMsg/6(ami_inspection)

== system VCU10/ESP ==
  note: 可不发
  ipc_esp_pressure : Inport
  brake_flag : Inport  Port=2
  canb_esp_t01 : Inport  Port=3
  canb_esp_t03 : Inport  Port=4
  canb_esp_t06 : Inport  Port=5
  canb_esp_t07 : Inport  Port=6
  function : TriggerPort  TriggerType=function-call  VariantControl=(inherit)
  ESP_ReceiveMsg : Subsystem
  ESP_TransmitMsg : Subsystem
  checkSum : Ground
  lifeSig : Ground
  canb_esp_r00 : Outport
  ESP_T_01sigal : Outport  Port=2
  ESP_T_03signal : Outport  Port=3
  ESP_T_06signal : Outport  Port=4
  ESP_T_07signal : Outport  Port=5
  brkmotor_check : Outport  Port=6
  wires:
  ESP_ReceiveMsg/5(brkmotor_check) -> brkmotor_check/1
  brake_flag/1 -> ESP_TransmitMsg/2(brake_flag)
  ipc_esp_pressure/1 -> ESP_TransmitMsg/1(ipc_esp_pressure)
  canb_esp_t01/1 -> ESP_ReceiveMsg/1(canb_esp_t01)
  canb_esp_t07/1 -> ESP_ReceiveMsg/4(canb_esp_t07)
  canb_esp_t06/1 -> ESP_ReceiveMsg/3(canb_esp_t06)
  canb_esp_t03/1 -> ESP_ReceiveMsg/2(canb_esp_t03)
  ESP_ReceiveMsg/1(ESP_T_01sigal) -> ESP_T_01sigal/1
  ESP_ReceiveMsg/4(ESP_T_07signal) -> ESP_T_07signal/1
  ESP_ReceiveMsg/3(ESP_T_06signal) -> ESP_T_06signal/1
  ESP_ReceiveMsg/2(ESP_T_03signal) -> ESP_T_03signal/1
  checkSum/1 -> ESP_TransmitMsg/4(checkSum)
  ESP_TransmitMsg/1(canb_esp_r00) -> canb_esp_r00/1
  lifeSig/1 -> ESP_TransmitMsg/3(lifeSig)

== system VCU10/IPC ==
  ipc_astask : Inport
  res_signal : Inport  Port=2
  canb_ipctsmsg1 : Inport  Port=3
  canb_ipctsmsg2 : Inport  Port=4
  steer_return : Inport  Port=5
  function : TriggerPort  TriggerType=function-call  VariantControl=(inherit)
  Bus Selector : BusSelector  OutputSignals=res_go,res_stop
  IPC_ReceiveMsg : Subsystem
  IPC_TransmitMsg : Subsystem
  ipc_esp_pressure : Outport
  ipc_motor_torque : Outport  Port=2
  ipc_eps_angle : Outport  Port=3
  ipc_eps_velocity : Outport  Port=4
  ipc_err : Outport  Port=5
  task_finish : Outport  Port=6
  ipc_heartbeat : Outport  Port=7
  ipc_lspd : Outport  Port=8
  ipc_hspd : Outport  Port=9
  canb_ipcrxmsg : Outport  Port=10
  wires:
  ipc_astask/1 -> IPC_ReceiveMsg/4(ipc_astask)
  res_signal/1 -> Bus Selector/1
  Bus Selector/1 -> IPC_ReceiveMsg/2(ipc_resgo)  "<res_go>"
  Bus Selector/2 -> IPC_ReceiveMsg/3(ipc_resstop)  "<res_stop>"
  IPC_TransmitMsg/6(task_finish) -> task_finish/1
  IPC_TransmitMsg/5(ipc_err) -> ipc_err/1
  IPC_TransmitMsg/4(ipc_eps_velocity) -> ipc_eps_velocity/1
  IPC_TransmitMsg/3(ipc_eps_angle) -> ipc_eps_angle/1
  IPC_TransmitMsg/2(ipc_motor_torque) -> ipc_motor_torque/1
  IPC_TransmitMsg/1(ipc_esp_pressure) -> ipc_esp_pressure/1
  canb_ipctsmsg2/1 -> IPC_TransmitMsg/2(canb_ipctsmsg2)
  canb_ipctsmsg1/1 -> IPC_TransmitMsg/1(canb_ipctsmsg1)
  IPC_ReceiveMsg/1(canb_ipcrxmsg) -> canb_ipcrxmsg/1
  IPC_TransmitMsg/7(ipc_heartbeat) -> ipc_heartbeat/1
  IPC_TransmitMsg/8(ipc_lspd) -> ipc_lspd/1
  IPC_TransmitMsg/9(ipc_hspd) -> ipc_hspd/1
  steer_return/1 -> IPC_ReceiveMsg/1(steer_return)

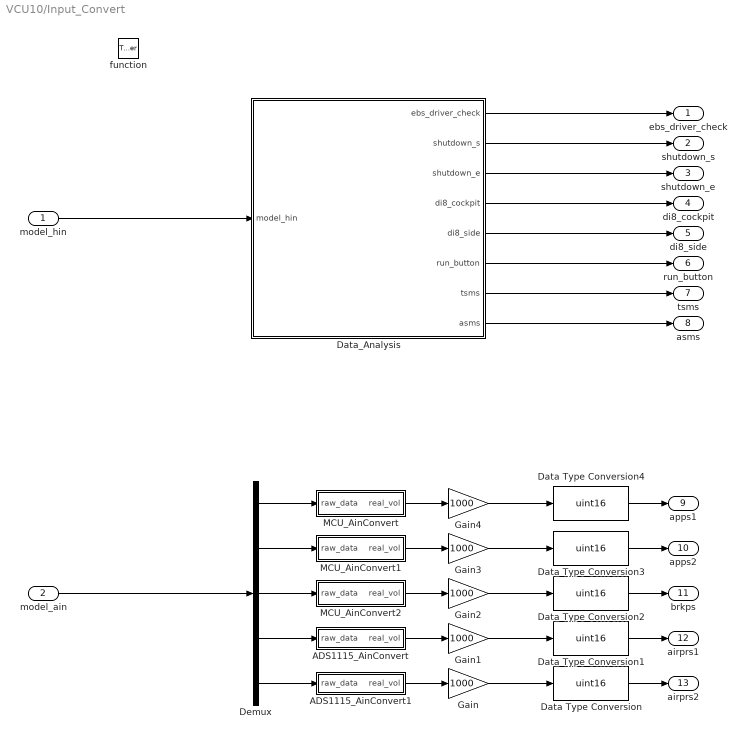
== system VCU10/Input_Convert ==
  model_hin : Inport
  model_ain : Inport  Port=2
  function : TriggerPort  TriggerType=function-call  VariantControl=(inherit)
  ADS1115_AinConvert : Subsystem
  ADS1115_AinConvert1 : Subsystem
  Data Type Conversion{,1..4} (5 alike) : DataTypeConversion  OutDataTypeStr=uint16
  Data_Analysis : Subsystem
  Demux : Demux  Outputs=5
  Gain{,1..4} (5 alike) : Gain  Gain=1000
  MCU_AinConvert : Subsystem
  MCU_AinConvert1 : Subsystem
  MCU_AinConvert2 : Subsystem
  ebs_driver_check : Outport
  shutdown_s : Outport  Port=2
  shutdown_e : Outport  Port=3
  di8_cockpit : Outport  Port=4
  di8_side : Outport  Port=5
  run_button : Outport  Port=6
  tsms : Outport  Port=7
  asms : Outport  Port=8
  apps1 : Outport  Port=9
  apps2 : Outport  Port=10
  brkps : Outport  Port=11
  airprs1 : Outport  Port=12
  airprs2 : Outport  Port=13
  wires:
  model_hin/1 -> Data_Analysis/1(model_hin)
  Data_Analysis/1(ebs_driver_check) -> ebs_driver_check/1
  Data_Analysis/2(shutdown_s) -> shutdown_s/1
  Data_Analysis/3(shutdown_e) -> shutdown_e/1
  Data_Analysis/4(di8_cockpit) -> di8_cockpit/1
  Data_Analysis/5(di8_side) -> di8_side/1
  Data_Analysis/6(run_button) -> run_button/1
  Data_Analysis/7(tsms) -> tsms/1
  Data_Analysis/8(asms) -> asms/1
  model_ain/1 -> Demux/1
  Demux/1 -> MCU_AinConvert/1(raw_data)
  Demux/2 -> MCU_AinConvert1/1(raw_data)
  Demux/3 -> MCU_AinConvert2/1(raw_data)
  Demux/4 -> ADS1115_AinConvert/1(raw_data)
  Demux/5 -> ADS1115_AinConvert1/1(raw_data)
  MCU_AinConvert/1(real_vol) -> Gain4/1
  MCU_AinConvert1/1(real_vol) -> Gain3/1
  MCU_AinConvert2/1(real_vol) -> Gain2/1
  ADS1115_AinConvert/1(real_vol) -> Gain1/1
  ADS1115_AinConvert1/1(real_vol) -> Gain/1
  Gain4/1 -> Data Type Conversion4/1
  Gain3/1 -> Data Type Conversion3/1
  Gain2/1 -> Data Type Conversion2/1
  Gain1/1 -> Data Type Conversion1/1
  Gain/1 -> Data Type Conversion/1
  Data Type Conversion4/1 -> apps1/1
  Data Type Conversion3/1 -> apps2/1
  Data Type Conversion2/1 -> brkps/1
  Data Type Conversion1/1 -> airprs1/1
  Data Type Conversion/1 -> airprs2/1

== system VCU10/LED_Control ==
  brake_on : Inport
  as_led_blue : Inport  Port=2
  as_led_yellow : Inport  Port=3
  asms_button : Inport  Port=4
  sensor_signal : Inport  Port=5
  res_stop : Inport  Port=6
  res_communication : Inport  Port=7
  Shutdown_Start : Inport  Port=8
  Shutdown_End : Inport  Port=9
  ESP_T_03signal : Inport  Port=10
  function : TriggerPort  TriggerType=function-call  VariantControl=(inherit)
  EBS_LED : Subsystem
  Subsystem : Subsystem
  Subsystem1 : Subsystem
  TSLED_Inspection : Stateflow chart  TreatAsAtomicUnit=on
  led_brake : Outport
  led_assi_blue : Outport  Port=2
  led_assi_yellow : Outport  Port=3
  led_ebs_error : Outport  Port=4
  led_imderr : Outport  Port=5
  led_bmserr : Outport  Port=6
  wires:
  brake_on/1 -> led_brake/1
  as_led_blue/1 -> Subsystem/1(as_led_blue)
  Subsystem/1(led_assi_blue) -> led_assi_blue/1
  Subsystem1/1(led_assi_yellow) -> led_assi_yellow/1
  as_led_yellow/1 -> Subsystem1/2(as_led_yellow)
  asms_button/1 -> Subsystem1/1(asms_button), [asms_button], Subsystem/2(asms_button)
  res_stop/1 -> EBS_LED/1(res_stop)
  res_communication/1 -> EBS_LED/2(res_communication)
  Shutdown_Start/1 -> EBS_LED/3(Shutdown_Start)
  Shutdown_End/1 -> EBS_LED/4(Shutdown_End)
  sensor_signal/1 -> EBS_LED/5(sensor_signal)
  ESP_T_03signal/1 -> EBS_LED/6(ESP_T_03signal)
  EBS_LED/1(led_ebs_error) -> led_ebs_error/1
  [asms_button] -> EBS_LED/7(asms_button)
  TSLED_Inspection/1(led_imderr) -> led_imderr/1
  TSLED_Inspection/2(led_bmserr) -> led_bmserr/1

== system VCU10/Motor_Control ==
  sensor_signal : Inport
  manual_driving_flag : Inport  Port=2
  as_flag : Inport  Port=3
  ipc_motor_torque : Inport  Port=4
  ts : Inport  Port=5
  function : TriggerPort  TriggerType=function-call  VariantControl=(inherit)
  ASTorque_Calculation : Subsystem
  MCU1_Rx_Command : Subsystem
  MCU1_Rx_Command3 : Subsystem
  ManualTorque_Calculation : Subsystem
  Motor_Torque_Stateflow : Stateflow chart  TreatAsAtomicUnit=on
      settings: PortSchema="{\"entries\":[{\"content\":{\"sides\":[{\"content\":{\"connectorIds\":[\"In1\",\"In3\",\"In2\",\"In4\"]},\"type\":\"ConnectorPlacement.EquallySpacedRectSide\",\"uuid\":\"d9a8263c-4b6f-42da-8ac2-d6351ac22d7e\"},{\"content\":{\"connectorIds\":[\"Out1\"],\"side\":\"RIGHT\"},\"type\":\"ConnectorPlacement.EquallySpacedRectSide\",\"uuid\":\"5afddd84-d4d9-4932-bab9-0cf7e7557aa2\"},{\"content\":{\"connectorIds\":[],\"side\":\"TOP\"},\"type\":\"ConnectorPlacement.EquallySpacedRectSide\",\"uuid\":\"31244ac9-97b6-45b3-a8be-c5389c850836\"}]},\"type\":\"ConnectorPlacement.EquallySpacedConnector\",\"uuid\":\"4a9ac252-b735-4ae7-9487-f10bc9e5bec6\"}],\"packageUris\":[\"http://schema.mathworks.com/mf0/Connector/R2020b\"],\"version\":\"1.0\"}"
  cana_motor_cmd : Outport
  cana_motor_cmd3 : Outport  Port=2
  wires:
  sensor_signal/1 -> ManualTorque_Calculation/1(sensor_signal)
  manual_driving_flag/1 -> Motor_Torque_Stateflow/1(manual_driving_flag)
  ManualTorque_Calculation/1(manual_torque) -> Motor_Torque_Stateflow/3(manual_torque)
  ASTorque_Calculation/1(as_torque) -> Motor_Torque_Stateflow/4(as_torque)
  Motor_Torque_Stateflow/1(motor_torque) -> [motor_torque]
  ts/1 -> MCU1_Rx_Command/1(ts)
  [motor_torque] -> MCU1_Rx_Command/2(motor_torque)
  MCU1_Rx_Command/1(cana_motor_cmd) -> cana_motor_cmd/1
  MCU1_Rx_Command3/1(cana_motor_cmd3) -> cana_motor_cmd3/1
  as_flag/1 -> Motor_Torque_Stateflow/2(as_task)
  ipc_motor_torque/1 -> ASTorque_Calculation/1(ipc_motor_torque)

== system VCU10/Output_Convert ==
  led_brake : Inport
  led_assi_y : Inport  Port=2
  led_assi_b : Inport  Port=3
  led_ebserror : Inport  Port=4
  res_error : Inport  Port=5
  ebs_trig : Inport  Port=6
  led_bmserr : Inport  Port=7
  led_imderr : Inport  Port=8
  di8 : Inport  Port=9
  run : Inport  Port=10
  buzzer_r2d : Inport  Port=11
  buzzer_ebs : Inport  Port=12
  function : TriggerPort  TriggerType=function-call  VariantControl=(inherit)
  Bit Concat : hdlsllib/Logic and Bit Operations/Bit Concat  numInputs=5
  Bit Concat1 : hdlsllib/Logic and Bit Operations/Bit Concat  numInputs=7
  model_lox : Outport
  model_hox : Outport  Port=2
  wires:
  res_error/1 -> Bit Concat/1
  led_ebserror/1 -> Bit Concat/2
  led_assi_b/1 -> Bit Concat/3
  led_assi_y/1 -> Bit Concat/4
  led_brake/1 -> Bit Concat/5
  Bit Concat/1 -> model_lox/1  "model_lox"
  di8/1 -> Bit Concat1/4
  led_imderr/1 -> Bit Concat1/5
  led_bmserr/1 -> Bit Concat1/6
  ebs_trig/1 -> Bit Concat1/7
  run/1 -> Bit Concat1/3
  buzzer_r2d/1 -> Bit Concat1/2
  buzzer_ebs/1 -> Bit Concat1/1
  Bit Concat1/1 -> model_hox/1  "model_hox"

== system VCU10/Res ==
  res_msg : Inport
  function : TriggerPort  TriggerType=function-call  VariantControl=(inherit)
  Bus Selector : BusSelector  OutputSignals=res_stop
  Res_Msg : Subsystem
  res_signal : Outport
  res_error : Outport  Port=2
  wires:
  res_msg/1 -> Res_Msg/1(res_msg)
  Res_Msg/1(res_signal) -> Bus Selector/1, res_signal/1
  Bus Selector/1 -> res_error/1  "<res_stop>"

== system VCU10/Sensor_Signal ==
  note: EBS气缸侧气压
  note: EBS气瓶侧气压
  apps1 : Inport
  apps2 : Inport  Port=2
  brkps : Inport  Port=3
  airprs_sensor1 : Inport  Port=4
  airprs_sensor2 : Inport  Port=5
  wlspd_fsensor : Inport  Port=6
  wlspd_hsensor : Inport  Port=7
  function : TriggerPort  TriggerType=function-call  VariantControl=(inherit)
  1-D Lookup Table : Lookup_n-D  NumberOfTableDimensions=1  BreakpointsForDimension1=[252 2000]  IndexSearchMethod=Linear search  Table=[0.0 1.0]  ExtrapMethod=Clip  UseLastTableValue=on  InternalRulePriority=Speed  OutDataTypeStr=double  RndMeth=Simplest  InputSameDT=on
  1-D Lookup Table1 : Lookup_n-D  NumberOfTableDimensions=1  BreakpointsForDimension1=[252 2000]  IndexSearchMethod=Linear search  Table=[0.0 1.0]  ExtrapMethod=Clip  UseLastTableValue=on  InternalRulePriority=Speed  OutDataTypeStr=double  RndMeth=Simplest  InputSameDT=on
  1-D Lookup Table9 : Lookup_n-D  NumberOfTableDimensions=1  BreakpointsForDimension1=[252 2000]  IndexSearchMethod=Linear search  Table=[0.0 1.0]  ExtrapMethod=Clip  UseLastTableValue=on  InternalRulePriority=Speed  OutDataTypeStr=double  RndMeth=Simplest  InputSameDT=on
  Bus Creator : BusCreator  Inputs=10
  Data Type Conversion{,1..9,12,15} (12 alike) : DataTypeConversion  OutDataTypeStr=double
  Gain : Gain  Gain=0.002
  Gain1 : Gain  Gain=0.002
  Saturation : Saturate  UpperLimit=1  LowerLimit=0
  Saturation1 : Saturate  UpperLimit=1  LowerLimit=0
  Saturation2 : Saturate  UpperLimit=1  LowerLimit=0
  Subsystem : Subsystem
  sensor_signal : Outport
  wires:
  apps1/1 -> Data Type Conversion1/1, 1-D Lookup Table/1
  1-D Lookup Table/1 -> Data Type Conversion/1
  Data Type Conversion/1 -> Saturation/1
  Saturation/1 -> Bus Creator/1  "apps1_01"
  Data Type Conversion1/1 -> Bus Creator/2  "apps1_raw"
  Data Type Conversion2/1 -> Saturation1/1
  apps2/1 -> 1-D Lookup Table9/1, Data Type Conversion3/1
  1-D Lookup Table9/1 -> Data Type Conversion2/1
  Saturation1/1 -> Bus Creator/3  "apps2_01"
  Data Type Conversion3/1 -> Bus Creator/4  "apps2_raw"
  brkps/1 -> 1-D Lookup Table1/1, Data Type Conversion5/1
  1-D Lookup Table1/1 -> Data Type Conversion4/1
  Data Type Conversion4/1 -> Saturation2/1
  Saturation2/1 -> Bus Creator/5  "brkps"
  Data Type Conversion5/1 -> Bus Creator/6  "brkps_raw"
  wlspd_fsensor/1 -> Data Type Conversion6/1
  Data Type Conversion6/1 -> Subsystem/1(f_frequency)
  wlspd_hsensor/1 -> Data Type Conversion7/1
  Data Type Conversion7/1 -> Subsystem/2(h_frequency)
  Subsystem/1(wheel_speed_f) -> Data Type Conversion8/1
  Subsystem/2(wheel_speed_h) -> Data Type Conversion9/1
  Data Type Conversion8/1 -> Bus Creator/7  "wlspd_fsensor"
  Data Type Conversion9/1 -> Bus Creator/8  "wlspd_hsensor"
  Bus Creator/1 -> sensor_signal/1
  Data Type Conversion12/1 -> Bus Creator/9  "airprs_sensor1"
  airprs_sensor2/1 -> Gain1/1
  Data Type Conversion15/1 -> Bus Creator/10  "airprs_sensor2"
  airprs_sensor1/1 -> Gain/1
  Gain/1 -> Data Type Conversion12/1
  Gain1/1 -> Data Type Conversion15/1
